simulink model "TwoLegRobotSim"  (R2022b)
settings: Solver=VariableStepAuto  StartTime=0.0  StopTime=10.0  MaxStep=1e-2  MinStep=1e-6  RelTol=1e-3
model workspace: external: MATLAB File D:\5720\Tutorial 2\TwoLegRobot_DataFile.m (data not in the file)
undefined symbols (not defined in the file): K, Mass_body, Mass_lower_leg, Mass_upper_leg, Mass_wheel, param_num, smiData, X, X_desired, Y, Z
libraries: sm_lib x73, nesl_utility x14, slpidlib x1
(part 1 of 3)
settings Model: Creator=Lyn20  LastModifiedBy=Lyn20

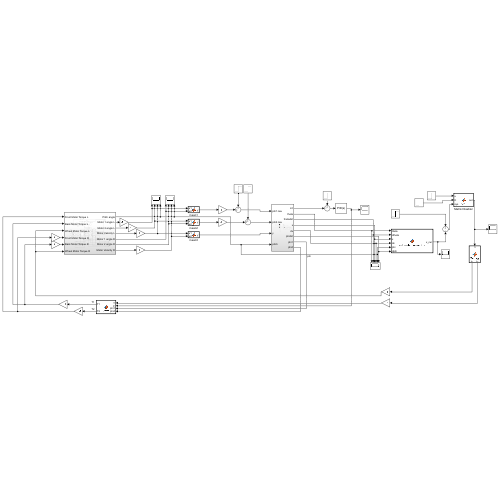
[thumbnail: Simulink's stored preview of the top-level diagram]
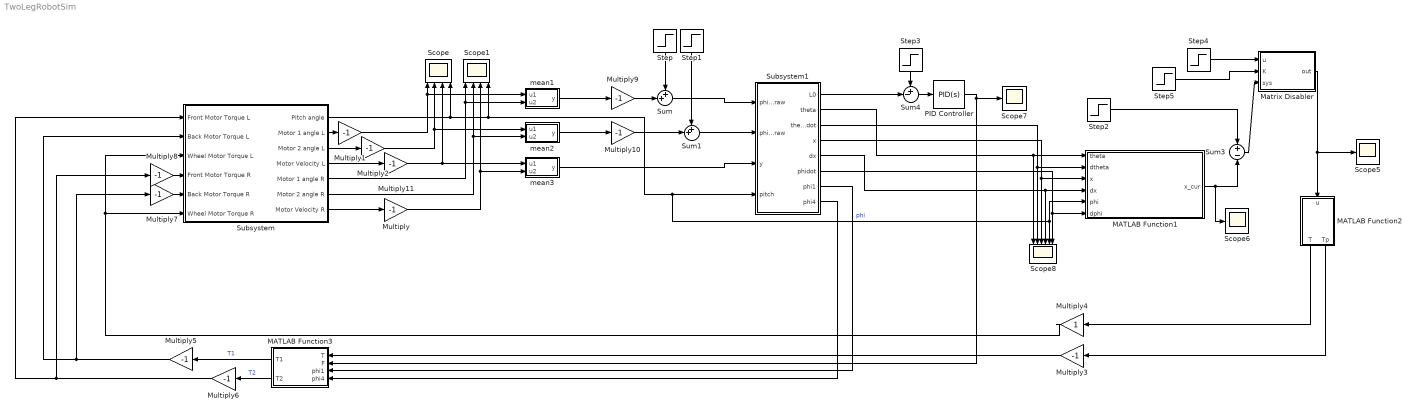
== system TwoLegRobotSim ==
  MATLAB Function1 : MATLAB Function  TreatAsAtomicUnit=on
  MATLAB Function2 : MATLAB Function  TreatAsAtomicUnit=on
  MATLAB Function3 : MATLAB Function  TreatAsAtomicUnit=on
  Matrix Disabler : MATLAB Function  TreatAsAtomicUnit=on
  Multiply{,1..3,5..11} (11 alike) : Gain  Gain=-1
  Multiply4 : Gain
  PID Controller : slpidlib/PID Controller  Controller=PID  Form=Parallel  TimeDomain=Continuous-time  UseExternalTs=off  SampleTime=0.01  IntegratorMethod=Forward Euler  FilterMethod=Forward Euler  ControllerParametersSource=internal  P=300  I=-1  UseKiTs=off  D=10  N=100  UseFilter=on  TunerSelectOption=Transfer Function Based (PID Tuner App)  InitialConditionSource=internal  InitialConditionForIntegrator=0  InitialConditionForFilter=0  DifferentiatorICPrevScaledInput=0  ExternalReset=none  TrackingMode=off  Kt=1  LimitOutput=off  SatLimitsSource=internal  UpperSaturationLimit=inf  LowerSaturationLimit=-inf  LinearizeAsGain=on  AntiWindupMode=none  Kb=1  LimitIntegrator=off  UpperIntegratorSaturationLimit=inf  LowerIntegratorSaturationLimit=-inf  POutMin=[]  POutMax=[]  IOutMin=[]  IOutMax=[]  DOutMin=[]  DOutMax=[]  NOutMin=[]  NOutMax=[]  SumOutMin=[]  SumOutMax=[]  SaturationOutMin=[]  SaturationOutMax=[]  PParamMin=[]  PParamMax=[]  IParamMin=[]  IParamMax=[]  DParamMin=[]  DParamMax=[]  NParamMin=[]  NParamMax=[]  KbParamMin=[]  KbParamMax=[]  KtParamMin=[]  KtParamMax=[]  KbOutMin=[]  KbOutMax=[]  KtOutMin=[]  KtOutMax=[]  IntegratorOutMin=[]  IntegratorOutMax=[]  FilterOutMin=[]  FilterOutMax=[]  SumI1OutMin=[]  SumI1OutMax=[]  SumI2OutMin=[]  SumI2OutMax=[]  SumI3OutMin=[]  SumI3OutMax=[]  SumI4OutMin=[]  SumI4OutMax=[]  SumDOutMin=[]  SumDOutMax=[]  DifferentiatorOutMin=[]  DifferentiatorOutMax=[]  FilterDiffOutCoefMin=[]  FilterDiffOutCoefMax=[]  ReciprocalOutMin=[]  ReciprocalOutMax=[]  SumDenOutMin=[]  SumDenOutMax=[]  SumNumOutMin=[]  SumNumOutMax=[]  DivideOutMin=[]  DivideOutMax=[]  UdiffTsProdOutMin=[]  UdiffTsProdOutMax=[]  NTsProdOutMin=[]  NTsProdOutMax=[]  UintegralTsProdOutMin=[]  UintegralTsProdOutMax=[]  UngainTsProdOutMin=[]  UngainTsProdOutMax=[]  ClampingZeroOutDataTypeStr=Inherit: Inherit via back propagation  ClampingZeroOutMin=[]  ClampingZeroOutMax=[]  FilterDenConstantOutDataTypeStr=Inherit: Inherit via back propagation  FilterDenConstantOutMin=[]  FilterDenConstantOutMax=[]  PCopyOutDataTypeStr=Inherit: Inherit via back propagation  PCopyOutMin=[]  PCopyOutMax=[]  NCopyOutDataTypeStr=Inherit: Inherit via back propagation  NCopyOutMin=[]  NCopyOutMax=[]  IntegratorContinuousStateAttributes=''  IntegratorStateMustResolveToSignalObject=off  IntegratorRTWStateStorageClass=Auto  FilterContinuousStateAttributes=''  FilterStateMustResolveToSignalObject=off  FilterRTWStateStorageClass=Auto  ParallelPVariant=InternalParameters  IdealPVariant=Disabled  IVariant=InternalParameters  DVariant=InternalParameters  IntegratorVariant=Continuous  SatVariant=Disabled  AWVariant=Passthrough  PCopyVariant=Disabled  TRVariant=Disabled  FdbkBlocksVariant=Forward  IdealPFdbkVariant=Disabled  SatFdbkVariant=Disabled  DerivativeFilterVariant=ContFilter  NVariant=InternalParameters  NCopyVariant=Disabled  FilterICVariant=InternalICsFilter  IntegratorICVariant=InternalICs  ExternalResetVariant=Disabled  TRSumVariant=Passthrough  SumFdbkVariant=Disabled  SumVariant=Sum_PID  TsampFilterVariant=InternalTs  TsampNgainVariant=Passthrough  TsampIntegralVariant=Passthrough  ExternalSaturationOutDataTypeStr=Inherit: Same as second input
  Scope : Scope  NumInputPorts=4
  Scope1 : Scope  NumInputPorts=4
  Scope5 : Scope
  Scope6 : Scope
  Scope7 : Scope
  Scope8 : Scope  NumInputPorts=6
  Step : Step  Time=0  After=1.5*pi  SampleTime=0
  Step1 : Step  Time=0  After=0.5*pi  SampleTime=0
  Step2 : Step  Time=1.5  Before=[0;X_desired;0;0;0;0]  After=[0;0;0;0;0;0]  SampleTime=0
  Step3 : Step  Time=0  After=param_num.L_m+param_num.L  SampleTime=0
  Step4 : Step  Time=0  SampleTime=0
  Step5 : Step  Time=0.2  After=K  SampleTime=0
  Subsystem : Subsystem
  Subsystem1 : Subsystem
  Sum : Sum  Inputs=++|
  Sum1 : Sum  Inputs=++|
  Sum3 : Sum  Inputs=+|-
  Sum4 : Sum  Inputs=+-|
  mean1 : MATLAB Function  TreatAsAtomicUnit=on
  mean2 : MATLAB Function  TreatAsAtomicUnit=on
  mean3 : MATLAB Function  TreatAsAtomicUnit=on
  wires:
  Subsystem/2(Motor 1 angle L) -> Multiply1/1
  Subsystem/3(Motor 2 angle L) -> Multiply2/1
  Subsystem/4(Motor Velocity L) -> Multiply11/1
  Subsystem1/1(L0) -> Sum4/2
  Subsystem1/6(phidot) -> Scope8/6, MATLAB Function1/6(dphi)
  Subsystem1/4(x) -> MATLAB Function1/3(x), Scope8/3
  MATLAB Function2/2(Tp) -> Multiply3/1
  Step4/1 -> Matrix Disabler/1(u)
  Multiply3/1 -> MATLAB Function3/1(T)
  Subsystem1/2(theta) -> MATLAB Function1/1(theta), Scope8/1
  Matrix Disabler/1(out) -> Scope5/1, MATLAB Function2/1(u)
  Subsystem1/5(dx) -> MATLAB Function1/4(dx), Scope8/4
  MATLAB Function2/1(T) -> Multiply4/1
  MATLAB Function1/1(x_cur) -> Scope6/1, Sum3/2
  Step5/1 -> Matrix Disabler/2(K)
  Subsystem/1(Pitch angle) -> Scope/4, Scope1/4, MATLAB Function1/5(phi), Scope8/5, Subsystem1/4(pitch)  "phi"
  Sum3/1 -> Matrix Disabler/3(sys)
  Sum4/1 -> PID Controller/1
  Step2/1 -> Sum3/1
  PID Controller/1 -> MATLAB Function3/2(F), Scope7/1
  Subsystem1/3(thetadot) -> Scope8/2, MATLAB Function1/2(dtheta)
  Step3/1 -> Sum4/1
  Multiply5/1 -> Multiply7/1, Subsystem/2(Back Motor Torque L)
  MATLAB Function3/2(T2) -> Multiply6/1  "T2"
  MATLAB Function3/1(T1) -> Multiply5/1  "T1"
  Subsystem1/8(phi4) -> MATLAB Function3/4(phi4)
  Subsystem1/7(phi1) -> MATLAB Function3/3(phi1)
  Subsystem/6(Motor 2 angle R) -> mean2/2(u2), Scope1/2
  Subsystem/7(Motor Velocity R) -> Multiply/1
  Subsystem/5(Motor 1 angle R) -> mean1/2(u2), Scope1/1
  Multiply/1 -> mean3/2(u2), Scope1/3
  Multiply1/1 -> mean1/1(u1), Scope/1
  Multiply2/1 -> mean2/1(u1), Scope/2
  mean1/1(y) -> Multiply9/1
  mean2/1(y) -> Multiply10/1
  Multiply6/1 -> Multiply8/1, Subsystem/1(Front Motor Torque L)
  Multiply9/1 -> Sum/2
  Sum/1 -> Subsystem1/1(phi1 raw)
  Multiply10/1 -> Sum1/2
  Sum1/1 -> Subsystem1/2(phi4 raw)
  Step/1 -> Sum/1
  Step1/1 -> Sum1/1
  Multiply8/1 -> Subsystem/4(Front Motor Torque R)
  Multiply7/1 -> Subsystem/5(Back Motor Torque R)
  Multiply4/1 -> Subsystem/6(Wheel Motor Torque R), Subsystem/3(Wheel Motor Torque L)
  Multiply11/1 -> Scope/3, mean3/1(u1)
  mean3/1(y) -> Subsystem1/3(y)
